simulink model "Project3_Part2_sim"  (R2018a)
settings: Solver=VariableStepAuto  StartTime=0.0  StopTime=10  FixedStep=.001  MaxStep=.001  RelTol=1e-6  EnableMultiTasking=on
values from neighbouring files (symbols this model uses):
  Kd = 350    [Project3_Part2.m]
  Kp = 3000    [Project3_Part2.m]
  trajectory = zeros(traj_mat_size(1)+1, traj_mat_size(2)+1)    [Project3_Part2.m]
(part 4 of 4)

== matlab function Project3_Part2_sim/MATLAB Function ==
  data: theta input; theta_ddot input; torque output; theta_dot input
function torque = newton_euler( theta, theta_ddot, theta_dot )
%#codegen
coder.extrinsic('evalin');
coder.extrinsic('newtonEuler');

persistent linkList boundry_conditions;

if isempty(linkList)
    linkList = evalin('base','linkList');
    boundry_conditions.base_angular_velocity = [0;0;0];
    boundry_conditions.base_angular_acceleration = [0;0;0];
    boundry_conditions.base_linear_acceleration = [0;0;9.8];
    boundry_conditions.distal_force = [0;0;0];
    boundry_conditions.distal_torque = [0;0;0];
end

% theta(2) = theta(2)-pi/2; % put in DH frame
torque = zeros(6,1);
torque = newtonEuler(linkList,theta,theta_dot,theta_ddot,boundry_conditions);


end

== matlab function Project3_Part2_sim/ABB Arm Dynamics/Laser Tracking ==
  data: theta input; pose output
function pose = laserTracker(theta)
%#codegen
coder.extrinsic('evalin');
persistent Sim_Exact;

if isempty(Sim_Exact)
    Sim_Exact = evalin('base','Sim_Exact');
end


th1 = theta(1);
th2 = theta(2);
th3 = theta(3);
th4 = theta(4);
th5 = theta(5);
th6 = theta(6);


if(Sim_Exact)
    pose = [ sin(th6)*(cos(th4)*sin(th1) + sin(th4)*(cos(th1)*sin(th2)*sin(th3) - cos(th1)*cos(th2)*cos(th3))) + cos(th6)*(cos(th5)*(sin(th1)*sin(th4) - cos(th4)*(cos(th1)*sin(th2)*sin(th3) - cos(th1)*cos(th2)*cos(th3))) - sin(th5)*(cos(th1)*cos(th2)*sin(th3) + cos(th1)*cos(th3)*sin(th2))), cos(th6)*(cos(th4)*sin(th1) + sin(th4)*(cos(th1)*sin(th2)*sin(th3) - cos(th1)*cos(th2)*cos(th3))) - sin(th6)*(cos(th5)*(sin(th1)*sin(th4) - cos(th4)*(cos(th1)*sin(th2)*sin(th3) - cos(th1)*cos(th2)*cos(th3))) - sin(th5)*(cos(th1)*cos(th2)*sin(th3) + cos(th1)*cos(th3)*sin(th2))), - sin(th5)*(sin(th1)*sin(th4) - cos(th4)*(cos(th1)*sin(th2)*sin(th3) - cos(th1)*cos(th2)*cos(th3))) - cos(th5)*(cos(th1)*cos(th2)*sin(th3) + cos(th1)*cos(th3)*sin(th2)), (27*cos(th1)*cos(th2))/100 - (9*sin(th5)*(sin(th1)*sin(th4) - cos(th4)*(cos(th1)*sin(th2)*sin(th3) - cos(th1)*cos(th2)*cos(th3))))/125 - (9*cos(th5)*(cos(th1)*cos(th2)*sin(th3) + cos(th1)*cos(th3)*sin(th2)))/125 - (7*cos(th1)*sin(th2)*sin(th3))/100 + (7*cos(th1)*cos(th2)*cos(th3))/100 - (151*cos(th1)*cos(th2)*sin(th3))/500 - (151*cos(th1)*cos(th3)*sin(th2))/500;
        - sin(th6)*(cos(th1)*cos(th4) - sin(th4)*(sin(th1)*sin(th2)*sin(th3) - cos(th2)*cos(th3)*sin(th1))) - cos(th6)*(cos(th5)*(cos(th1)*sin(th4) + cos(th4)*(sin(th1)*sin(th2)*sin(th3) - cos(th2)*cos(th3)*sin(th1))) + sin(th5)*(cos(th2)*sin(th1)*sin(th3) + cos(th3)*sin(th1)*sin(th2))), sin(th6)*(cos(th5)*(cos(th1)*sin(th4) + cos(th4)*(sin(th1)*sin(th2)*sin(th3) - cos(th2)*cos(th3)*sin(th1))) + sin(th5)*(cos(th2)*sin(th1)*sin(th3) + cos(th3)*sin(th1)*sin(th2))) - cos(th6)*(cos(th1)*cos(th4) - sin(th4)*(sin(th1)*sin(th2)*sin(th3) - cos(th2)*cos(th3)*sin(th1))), sin(th5)*(cos(th1)*sin(th4) + cos(th4)*(sin(th1)*sin(th2)*sin(th3) - cos(th2)*cos(th3)*sin(th1))) - cos(th5)*(cos(th2)*sin(th1)*sin(th3) + cos(th3)*sin(th1)*sin(th2)), (27*cos(th2)*sin(th1))/100 + (9*sin(th5)*(cos(th1)*sin(th4) + cos(th4)*(sin(th1)*sin(th2)*sin(th3) - cos(th2)*cos(th3)*sin(th1))))/125 - (9*cos(th5)*(cos(th2)*sin(th1)*sin(th3) + cos(th3)*sin(th1)*sin(th2)))/125 - (151*cos(th2)*sin(th1)*sin(th3))/500 - (151*cos(th3)*sin(th1)*sin(th2))/500 - (7*sin(th1)*sin(th2)*sin(th3))/100 + (7*cos(th2)*cos(th3)*sin(th1))/100;
        sin(th4)*sin(th6)*(cos(th2)*sin(th3) + cos(th3)*sin(th2)) - cos(th6)*(sin(th5)*(cos(th2)*cos(th3) - sin(th2)*sin(th3)) + cos(th4)*cos(th5)*(cos(th2)*sin(th3) + cos(th3)*sin(th2))), sin(th6)*(sin(th5)*(cos(th2)*cos(th3) - sin(th2)*sin(th3)) + cos(th4)*cos(th5)*(cos(th2)*sin(th3) + cos(th3)*sin(th2))) + cos(th6)*sin(th4)*(cos(th2)*sin(th3) + cos(th3)*sin(th2)), cos(th4)*sin(th5)*(cos(th2)*sin(th3) + cos(th3)*sin(th2)) - cos(th5)*(cos(th2)*cos(th3) - sin(th2)*sin(th3)), (151*sin(th2)*sin(th3))/500 - (151*cos(th2)*cos(th3))/500 - (7*cos(th2)*sin(th3))/100 - (7*cos(th3)*sin(th2))/100 - (27*sin(th2))/100 - (9*cos(th5)*(cos(th2)*cos(th3) - sin(th2)*sin(th3)))/125 + (9*cos(th4)*sin(th5)*(cos(th2)*sin(th3) + cos(th3)*sin(th2)))/125 + 29/100;
        0, 0, 0, 1];
else
    
    pose = [ sin(th6)*(cos(th4)*sin(th1) + sin(th4)*(cos(th1)*sin(th2)*sin(th3) - cos(th1)*cos(th2)*cos(th3))) + cos(th6)*(cos(th5)*(sin(th1)*sin(th4) - cos(th4)*(cos(th1)*sin(th2)*sin(th3) - cos(th1)*cos(th2)*cos(th3))) - sin(th5)*(cos(th1)*cos(th2)*sin(th3) + cos(th1)*cos(th3)*sin(th2))), cos(th6)*(cos(th4)*sin(th1) + sin(th4)*(cos(th1)*sin(th2)*sin(th3) - cos(th1)*cos(th2)*cos(th3))) - sin(th6)*(cos(th5)*(sin(th1)*sin(th4) - cos(th4)*(cos(th1)*sin(th2)*sin(th3) - cos(th1)*cos(th2)*cos(th3))) - sin(th5)*(cos(th1)*cos(th2)*sin(th3) + cos(th1)*cos(th3)*sin(th2))), - sin(th5)*(sin(th1)*sin(th4) - cos(th4)*(cos(th1)*sin(th2)*sin(th3) - cos(th1)*cos(th2)*cos(th3))) - cos(th5)*(cos(th1)*cos(th2)*sin(th3) + cos(th1)*cos(th3)*sin(th2)), (151838081588107*cos(th1)*cos(th2))/562949953421312 - (123928564092639*sin(th1))/72057594037927936 - (7184037743251309*cos(th1))/36893488147419103232 - (7330531551818703*cos(th4)*sin(th1))/36893488147419103232 - (5489399374888815*sin(th1)*sin(th4))/9223372036854775808 + (970893499285375*cos(th5)*(sin(th1)*sin(th4) - cos(th4)*(cos(th1)*sin(th2)*sin(th3) - cos(th1)*cos(th2)*cos(th3))))/9223372036854775808 - (5192391675427195*sin(th5)*(sin(th1)*sin(th4) - cos(th4)*(cos(th1)*sin(th2)*sin(th3) - cos(th1)*cos(th2)*cos(th3))))/72057594037927936 + (1663072680156839*sin(th6)*(cos(th4)*sin(th1) + sin(th4)*(cos(th1)*sin(th2)*sin(th3) - cos(th1)*cos(th2)*cos(th3))))/2305843009213693952 + (1663072680156839*cos(th6)*(cos(th5)*(sin(th1)*sin(th4) - cos(th4)*(cos(th1)*sin(th2)*sin(th3) - cos(th1)*cos(th2)*cos(th3))) - sin(th5)*(cos(th1)*cos(th2)*sin(th3) + cos(th1)*cos(th3)*sin(th2))))/2305843009213693952 + (5489399374888815*cos(th4)*(cos(th1)*sin(th2)*sin(th3) - cos(th1)*cos(th2)*cos(th3)))/9223372036854775808 - (5192391675427195*cos(th5)*(cos(th1)*cos(th2)*sin(th3) + cos(th1)*cos(th3)*sin(th2)))/72057594037927936 - (7330531551818703*sin(th4)*(cos(th1)*sin(th2)*sin(th3) - cos(th1)*cos(th2)*cos(th3)))/36893488147419103232 - (970893499285375*sin(th5)*(cos(th1)*cos(th2)*sin(th3) + cos(th1)*cos(th3)*sin(th2)))/9223372036854775808 - (1259578569946919*cos(th1)*sin(th2)*sin(th3))/18014398509481984 + (1259578569946919*cos(th1)*cos(th2)*cos(th3))/18014398509481984 - (5430591396830085*cos(th1)*cos(th2)*sin(th3))/18014398509481984 - (5430591396830085*cos(th1)*cos(th3)*sin(th2))/18014398509481984;
        - sin(th6)*(cos(th1)*cos(th4) - sin(th4)*(sin(th1)*sin(th2)*sin(th3) - cos(th2)*cos(th3)*sin(th1))) - cos(th6)*(cos(th5)*(cos(th1)*sin(th4) + cos(th4)*(sin(th1)*sin(th2)*sin(th3) - cos(th2)*cos(th3)*sin(th1))) + sin(th5)*(cos(th2)*sin(th1)*sin(th3) + cos(th3)*sin(th1)*sin(th2))), sin(th6)*(cos(th5)*(cos(th1)*sin(th4) + cos(th4)*(sin(th1)*sin(th2)*sin(th3) - cos(th2)*cos(th3)*sin(th1))) + sin(th5)*(cos(th2)*sin(th1)*sin(th3) + cos(th3)*sin(th1)*sin(th2))) - cos(th6)*(cos(th1)*cos(th4) - sin(th4)*(sin(th1)*sin(th2)*sin(th3) - cos(th2)*cos(th3)*sin(th1))), sin(th5)*(cos(th1)*sin(th4) + cos(th4)*(sin(th1)*sin(th2)*sin(th3) - cos(th2)*cos(th3)*sin(th1))) - cos(th5)*(cos(th2)*sin(th1)*sin(th3) + cos(th3)*sin(th1)*sin(th2)), (123928564092639*cos(th1))/72057594037927936 - (7184037743251309*sin(th1))/36893488147419103232 + (7330531551818703*cos(th1)*cos(th4))/36893488147419103232 + (151838081588107*cos(th2)*sin(th1))/562949953421312 + (5489399374888815*cos(th1)*sin(th4))/9223372036854775808 - (970893499285375*cos(th5)*(cos(th1)*sin(th4) + cos(th4)*(sin(th1)*sin(th2)*sin(th3) - cos(th2)*cos(th3)*sin(th1))))/9223372036854775808 + (5192391675427195*sin(th5)*(cos(th1)*sin(th4) + cos(th4)*(sin(th1)*sin(th2)*sin(th3) - cos(th2)*cos(th3)*sin(th1))))/72057594037927936 - (1663072680156839*sin(th6)*(cos(th1)*cos(th4) - sin(th4)*(sin(th1)*sin(th2)*sin(th3) - cos(th2)*cos(th3)*sin(th1))))/2305843009213693952 + (5489399374888815*cos(th4)*(sin(th1)*sin(th2)*sin(th3) - cos(th2)*cos(th3)*sin(th1)))/9223372036854775808 - (5192391675427195*cos(th5)*(cos(th2)*sin(th1)*sin(th3) + cos(th3)*sin(th1)*sin(th2)))/72057594037927936 - (1663072680156839*cos(th6)*(cos(th5)*(cos(th1)*sin(th4) + cos(th4)*(sin(th1)*sin(th2)*sin(th3) - cos(th2)*cos(th3)*sin(th1))) + sin(th5)*(cos(th2)*sin(th1)*sin(th3) + cos(th3)*sin(th1)*sin(th2))))/2305843009213693952 - (7330531551818703*sin(th4)*(sin(th1)*sin(th2)*sin(th3) - cos(th2)*cos(th3)*sin(th1)))/36893488147419103232 - (970893499285375*sin(th5)*(cos(th2)*sin(th1)*sin(th3) + cos(th3)*sin(th1)*sin(th2)))/9223372036854775808 - (5430591396830085*cos(th2)*sin(th1)*sin(th3))/18014398509481984 - (5430591396830085*cos(th3)*sin(th1)*sin(th2))/18014398509481984 - (1259578569946919*sin(th1)*sin(th2)*sin(th3))/18014398509481984 + (1259578569946919*cos(th2)*cos(th3)*sin(th1))/18014398509481984;
        sin(th4)*sin(th6)*(cos(th2)*sin(th3) + cos(th3)*sin(th2)) - cos(th6)*(sin(th5)*(cos(th2)*cos(th3) - sin(th2)*sin(th3)) + cos(th4)*cos(th5)*(cos(th2)*sin(th3) + cos(th3)*sin(th2))), sin(th6)*(sin(th5)*(cos(th2)*cos(th3) - sin(th2)*sin(th3)) + cos(th4)*cos(th5)*(cos(th2)*sin(th3) + cos(th3)*sin(th2))) + cos(th6)*sin(th4)*(cos(th2)*sin(th3) + cos(th3)*sin(th2)), cos(th4)*sin(th5)*(cos(th2)*sin(th3) + cos(th3)*sin(th2)) - cos(th5)*(cos(th2)*cos(th3) - sin(th2)*sin(th3)), (5430591396830085*sin(th2)*sin(th3))/18014398509481984 - (5430591396830085*cos(th2)*cos(th3))/18014398509481984 - (1259578569946919*cos(th2)*sin(th3))/18014398509481984 - (1259578569946919*cos(th3)*sin(th2))/18014398509481984 - (1663072680156839*cos(th6)*(sin(th5)*(cos(th2)*cos(th3) - sin(th2)*sin(th3)) + cos(th4)*cos(th5)*(cos(th2)*sin(th3) + cos(th3)*sin(th2))))/2305843009213693952 - (151838081588107*sin(th2))/562949953421312 + (5489399374888815*cos(th4)*(cos(th2)*sin(th3) + cos(th3)*sin(th2)))/9223372036854775808 - (5192391675427195*cos(th5)*(cos(th2)*cos(th3) - sin(th2)*sin(th3)))/72057594037927936 - (7330531551818703*sin(th4)*(cos(th2)*sin(th3) + cos(th3)*sin(th2)))/36893488147419103232 - (970893499285375*sin(th5)*(cos(th2)*cos(th3) - sin(th2)*sin(th3)))/9223372036854775808 - (970893499285375*cos(th4)*cos(th5)*(cos(th2)*sin(th3) + cos(th3)*sin(th2)))/9223372036854775808 + (5192391675427195*cos(th4)*sin(th5)*(cos(th2)*sin(th3) + cos(th3)*sin(th2)))/72057594037927936 + (1663072680156839*sin(th4)*sin(th6)*(cos(th2)*sin(th3) + cos(th3)*sin(th2)))/2305843009213693952 + 325695105792877/1125899906842624;
        0, 0, 0, 1];
end

== matlab function Project3_Part2_sim/MATLAB Function1 ==
  data: t input; pos_des output; pos_dd_des output; pos_d_des output; trajectory input
%   Interp_Target provides the position (p), velocity (v), and
%   acceleration (a) at time t for a trajectory interpolated using the 
%   constant acceleration approach. Each of these are length M vectors. In
%   this case, we are interpolating [x;y;z;Q] (where Q is the quaternion 
%   values of xyz) into desired position, velocity, and acceleration in
%   operational & quaternion space.
% 
%   pos_des = the position at time t for a trajectory interpolated using the 
%   constant acceleration approach.
%   pos_d_des = the velocity at time t for a trajectory interpolated using the 
%   constant acceleration approach.
%   pos_dd_des = the acceleration at time t for a trajectory interpolated using the 
%   constant acceleration approach.
%   
%   t = the time of interest (these will be evenly spaced)
%   trajectory = a Nx(M+1) array of points. There are N waypoints in the 
%   trajectory of dimension M. The first column is the time for each point 
%   in the trajectory and the remaining M columns are the point to be 
%   reached at that time. 
%   transPercent = The percentage of the trajectory time to use for the 
%   constant acceleration transition. This must be in the range [0, 0.5]
%
%   Casey Duncan
%   10834922
%   MEGN 544
%   12/12/2018

function [pos_des, pos_dd_des, pos_d_des] = Interp_Target(t, trajectory)
    n = length(trajectory(:,1));
    num_x = length(trajectory(1,2:end));
    
    % Pre-allocate all vector variables
    pos_des = zeros(7,1);
    pos_d_des = zeros(6,1);
    pos_dd_des = zeros(6,1);
    
    p = zeros(7,1);
    v = zeros(7,1);
    a = zeros(7,1);
    
    x_des = zeros(3,1);
    x_d_des = zeros(3,1);
    x_dd_des = zeros(3,1);
    
    Q_des = zeros(4,1);
    Q_d_des = zeros(3,1);
    Q_dd_des = zeros(3,1);
    
    % Define tau:
    transPercent = 0.01;
    tau = transPercent;
    
    % Define trajectory times and position values
    t_traj = trajectory(:,1);
    pos = trajectory(:,2:end);
    
    t_end = t_traj(n);
    % Run Constant Acceleration Interpolation:
    if t > t_end
        p = pos(end,1:end)';
        v = zeros(num_x,1);
    else    
        for j = 2:(n-1)
                P0_all_th = pos(j-1,:);
                P1_all_th = pos(j,:);
                P2_all_th = pos(j+1,:);
                t0 = t_traj(j-1);
                t1 = t_traj(j);
                t2 = t_traj(j+1);

                % Const Accel: (0 <= t < tau) seconds
                if (j-1) == 1 && t >= t0 && t <= t0+tau
                    for k = 1:num_x
                        P1 = P0_all_th(k);
                        P2 = P1_all_th(k);
                        dP2 = P2-P1;
                        t2 = t_traj(j);
                        t1 = t_traj(j-1);

                        p(k,1) = P1+(dP2/(4*tau*(t2-t1)))*(t-t1+tau)^2;
                        v(k,1) = (dP2/(2*tau*(t2-t1)))*(t-t1+tau);
                        a(k,1) = 2*dP2/(4*tau*(t2-t1));
                    end

                    break;
                    
                % Const Accel: (t_end-tau <= t < t_end) seconds
                elseif j+1 == n && t >= t2-tau && t <= t2
                    for k = 1:num_x
                        P0 = P1_all_th(k);
                        P1 = P2_all_th(k);
                        dP1 = P1-P0;
                        t0 = t_traj(j);
                        t1 = t_traj(j+1);

                        p(k,1) = P1-(dP1/(4*tau*(t1-t0)))*(t-t1-tau)^2;
                        v(k,1) = -(dP1/(2*tau*(t1-t0)))*(t-t1-tau);
                        a(k,1) = -2*dP1/(4*tau*(t1-t0));
                    end
                    break;
                    
                % Const +Vel: (tau <= t < t_end-tau) seconds    
                elseif t >= t0+tau && t <= t1-tau
                    for k = 1:num_x
                        P0 = P0_all_th(k);
                        P1 = P1_all_th(k);
                        dP1 = P1-P0;

                        p(k,1) = P1-((t1-t)/(t1-t0))*dP1;
                        v(k,1) = dP1/(t1-t0);
                        a(k,1) = 0;
                    end
                    break;

                % Const Acc: (tau <= t < t_end-tau) seconds    
                elseif t >= t1-tau && t <= t1+tau
                    for k = 1:num_x
                        P0 = P0_all_th(k);
                        P1 = P1_all_th(k);
                        P2 = P2_all_th(k);
                        dP1 = P1-P0;
                        dP2 = P2-P1;

                        p(k,1) = P1-(dP1/(4*tau*(t1-t0)))*(t-t1-tau)^2+(dP2/(4*tau*(t2-t1)))*(t-t1+tau)^2;
                        v(k,1) = -(dP1/(2*tau*(t1-t0)))*(t-t1-tau)+(dP2/(2*tau*(t2-t1)))*(t-t1+tau);
                        a(k,1) = -2*dP1/(4*tau*(t1-t0))+2*dP2/(4*tau*(t2-t1)); 
                    end
                    break;

                % Const -Vel: (tau <= t < t_end-tau) seconds    
                elseif t >= t1+tau && t <= t2-tau
                    for k = 1:num_x
                        P1 = P1_all_th(k);
                        P2 = P2_all_th(k);
                        dP2 = P2-P1;

                        p(k,1) = P1+((t-t1)/(t2-t1))*dP2;
                        v(k,1) = dP2/(t2-t1);
                        a(k,1) = 0; 
                    end
                    break;

                end
        end
    end
       
    % Assign output values
    x_des = p(1:3,1);
    x_d_des = v(1:3,1);
    x_dd_des = a(1:3,1);
    
    Q_des = p(4:end,1);
    q_0 = Q_des(1);
    q = Q_des(2:end);
    Q_d_des = 2*[-q, (q_0*eye(3))+cpMap(q)]*v(4:end,1);
    Q_dd_des = 2*[-q, (q_0*eye(3))+cpMap(q)]*a(4:end,1);
    
    pos_des = [x_des; Q_des];
    pos_d_des = [x_d_des; Q_d_des];
    pos_dd_des = [x_dd_des; Q_dd_des];
end

== matlab function Project3_Part2_sim/MATLAB Function2 ==
  data: T_act output; paramList input
%   FwdKine_Actual returns the homeogenious transformation matrix of the
%   robot manipulator in its current position
% 
%   T_act = forward kinematics of a manipulator with the provided DH 
%   parameter set.
%   
%   linkList = an array of links, each created by createLink (Provided by
%   Geometry function).
%   paramList = an array containing the current state of their joint 
%   variables.
%
%   Casey Duncan
%   10834922
%   MEGN 544
%   12/12/2018

function T_act  = FwdKine_Actual(paramList)
    % Geometry Function:
    % ABB Geometry
    d1 = 0.29;
    a2 = 0.270;
    a3 = 0.070;
    d4 = 0.302;
    d6 = 0.072;

    rcom1 = [0;-d1/2;0];
    rcom2 = [-a2/2;0;0];
    rcom3 = [-a3/2;0;0];
    rcom4 = [0;-d4/2;0];
    rcom5 = [0;0;0];
    rcom6 = [0; -d6/2;0];

    rad1 = .2/2; h1 = d1;   m1 = 8050*h1*rad1^2*pi;
    rad2 = .15/2; h2 = a2;   m2 = 8050*h2*rad2^2*pi;
    rad3 = .1/2; h3 = a3;  m3 = 8050*h3*rad3^2*pi;
    rad4 = .1/2; h4 = d4;  m4 = 8050*h4*rad4^2*pi;
    rad5 = .05/2; h5 = .125; m5 = 8050*h5*rad5^2*pi;
    rad6 = .05/2; h6 = d6;  m6 = 8050*h6*rad6^2*pi;

    J1 = diag(m1*[1/12*(3*rad1^2+h1^2),rad1^2/2,1/12*(3*rad1^2+h1^2)]);
    J2 = diag(m2*[rad2^2/2,1/12*(3*rad2^2+h2^2),1/12*(3*rad2^2+h2^2)]);
    J3 = diag(m3*[rad3^2/2,1/12*(3*rad3^2+h3^2),1/12*(3*rad3^2+h3^2)]);
    J4 = diag(m4*[1/12*(3*rad4^2+h4^2),rad4^2/2,1/12*(3*rad4^2+h4^2)]);
    J5 = diag(m5*[1/12*(3*rad5^2+h5^2),rad5^2/2,1/12*(3*rad5^2+h5^2)]);
    J6 = diag(m6*[1/12*(3*rad6^2+h6^2),rad6^2/2,1/12*(3*rad6^2+h6^2)]);

    L1 = createLink(0,d1,-pi/2,[],rcom1, m1,J1);
    L2 = createLink(a2,0,0,[],rcom2, m2,J2);
    L3 = createLink(a3,0,-pi/2,[],rcom3, m3,J3);
    L4 = createLink(0,d4,pi/2,[],rcom4, m4,J4);
    L5 = createLink(0,0,-pi/2,[],rcom5, m5,J5);
    L6 = createLink(0,d6,0,[],rcom6, m6,J6);

    linkList = [L1;L2;L3;L4;L5;L6];

    % dhFwdKine Function
    % Preallocate output:
    T_act = zeros(4,4);
    
    Link_qty = length(linkList);
    T = eye(4);
    
    for i = 1:Link_qty
        L_i = linkList(i);
        
        % If link is Rotary, use theta from paramList:
            th_i = paramList(i);
            T_i = dhTransform(L_i.a, L_i.d, L_i.alpha, th_i);
        
        
        % Calculate transformation matrix (T_0,N) for manipulator from 
        % world frame to end effector
        T = T*T_i;
    end
    
    % The forward kinematics for the manipulator is just 
    T_act = T;
    
end

== matlab function Project3_Part2_sim/MATLAB Function3 ==
  data: T_act input; pos_des input; x_err output
%   x_err returns a 6x1 vector, where the first 3 elements 
%   are position error (desired - current), and the last three elements are 
%   an angle-axis representation of rotation error. Both expressed in the 
%   shared base frame.  
% 
%   error_vector = a 6x1 vector describing the error 
%   ([pos_error;rot_error]) as expressed in the shared base frame.
%   
%   pos_des = the vector [xyz; quaternion] describing the coordinate pose 
%   of the robot in XYZ & quaternion space ([xyz; quaternion]) in the 
%   reference frame (of the world for example).
%   T_act = the homogenious matrix describing the current coordinate frame 
%   (of the robot for example) in the reference frame (of the world for 
%   example).
%
%   Casey Duncan
%   10834922
%   MEGN 544
%   12/12/2018
%
function x_err = x_err(T_act, pos_des)
    x_err = zeros(6,1);

    x_des = pos_des(1:3,1);
    Q_des = pos_des(4:end,1);
    q_0 = Q_des(1);
    q = Q_des(2:end);
    
    % Use Quat2Rot to conver quaternion to rotation matrix:
    R_des = (q_0^2-(q.')*q)*eye(3)+2*q_0*cpMap(q)+2*(q*q.');
    
    % Use rotation matrix with xyz vals to make desired tranfromation
    % matrix:
    T_des = [R_des, x_des; 0, 0, 0, 1];
    
    % Implement TransErr to find x_err
    d_d = T_des(1:3,4);
    d_c = T_act(1:3,4);
    
    x_err(1:3,1) = d_d-d_c;
    
    rot_error_vector = rotationError(R_des, T_act(1:3,1:3));
    x_err(4:end,1) = rot_error_vector;
    
end

== matlab function Project3_Part2_sim/MATLAB Function4 ==
  data: Jv_inv_act output; pos_dd_act output; Theta_d_act input; Theta_act input; pos_d_act output
%   velJac_Actual returns the velocity jacobian of the manipulator
%   given an array of links created by the createLink function and the 
%   current joint variables. This is then used to calculate the desired
%   velocity & acceleration of the manipulator.
% 
%   Jv_inv_act = inverse of velocity jacobian
%   pos_d_act = desired velocity of the manipulator
%   pos_dd_act = desired acceleration of the manipulator
%   
%   linkList = the list of joint parameters created with createLink (this
%   comes from the geometry function)
%   Theta_act = the current theta for the joints. (an Nx1 array)
%   Theta_d_act = the current theta_dot values for the joints. 
%   (an Nx1 array)
%
%   Casey Duncan
%   10834922
%   MEGN 544
%   12/12/2018
%
function [Jv_inv_act, pos_dd_act, pos_d_act]  = velJac_Actual(Theta_d_act, Theta_act)
    % Geometry Function:
    % ABB Geometry
    d1 = 0.29;
    a2 = 0.270;
    a3 = 0.070;
    d4 = 0.302;
    d6 = 0.072;

    rcom1 = [0;-d1/2;0];
    rcom2 = [-a2/2;0;0];
    rcom3 = [-a3/2;0;0];
    rcom4 = [0;-d4/2;0];
    rcom5 = [0;0;0];
    rcom6 = [0; -d6/2;0];

    rad1 = .2/2; h1 = d1;   m1 = 8050*h1*rad1^2*pi;
    rad2 = .15/2; h2 = a2;   m2 = 8050*h2*rad2^2*pi;
    rad3 = .1/2; h3 = a3;  m3 = 8050*h3*rad3^2*pi;
    rad4 = .1/2; h4 = d4;  m4 = 8050*h4*rad4^2*pi;
    rad5 = .05/2; h5 = .125; m5 = 8050*h5*rad5^2*pi;
    rad6 = .05/2; h6 = d6;  m6 = 8050*h6*rad6^2*pi;

    J1 = diag(m1*[1/12*(3*rad1^2+h1^2),rad1^2/2,1/12*(3*rad1^2+h1^2)]);
    J2 = diag(m2*[rad2^2/2,1/12*(3*rad2^2+h2^2),1/12*(3*rad2^2+h2^2)]);
    J3 = diag(m3*[rad3^2/2,1/12*(3*rad3^2+h3^2),1/12*(3*rad3^2+h3^2)]);
    J4 = diag(m4*[1/12*(3*rad4^2+h4^2),rad4^2/2,1/12*(3*rad4^2+h4^2)]);
    J5 = diag(m5*[1/12*(3*rad5^2+h5^2),rad5^2/2,1/12*(3*rad5^2+h5^2)]);
    J6 = diag(m6*[1/12*(3*rad6^2+h6^2),rad6^2/2,1/12*(3*rad6^2+h6^2)]);

    L1 = createLink(0,d1,-pi/2,[],rcom1, m1,J1);
    L2 = createLink(a2,0,0,[],rcom2, m2,J2);
    L3 = createLink(a3,0,-pi/2,[],rcom3, m3,J3);
    L4 = createLink(0,d4,pi/2,[],rcom4, m4,J4);
    L5 = createLink(0,0,-pi/2,[],rcom5, m5,J5);
    L6 = createLink(0,d6,0,[],rcom6, m6,J6);

    linkList = [L1;L2;L3;L4;L5;L6];
    
    % Vel Jac Function:
    pos_d_act = zeros(6,1);
    pos_dd_act = zeros(6,1);
    Jv_inv_act = zeros(6,6);
    
    Jv = zeros(6,6);
    JvDot = zeros(6,6);
    
    paramList = Theta_act;
    paramRateList = Theta_d_act;
    
    [Jv, JvDot] = velocityJacobian(linkList, paramList, paramRateList) ;
       
    pos_d_act = Jv*Theta_d_act;
    pos_dd_act = JvDot*Theta_d_act;
    Jv_inv_act = pinv(Jv);

end

== matlab function Project3_Part2_sim/MATLAB Function5 ==
  data: x_dd_cont input; Jv_inv_act input; th_dd_cont output
%   Theta_dd_act returns the homeogenious transformation matrix of the
%   robot manipulator in its current position
% 
%   x_dd_cont = control acceleration.
%   Jv_inv_act = inverse of the jacobian matrix
%   
%   th_dd_cont = outputs joint acceleration control
%
%   Casey Duncan
%   10834922
%   MEGN 544
%   12/12/2018

function th_dd_cont = Theta_dd_act(x_dd_cont, Jv_inv_act)
    
    % Preallocate output
    th_dd_cont = zeros(6,1);
    th_dd_cont = Jv_inv_act*x_dd_cont;
end
